simulink model "sym_model copia"  (R2024b)
settings: Solver=FixedStepAuto  StartTime=0  StopTime=24*3600  FixedStep=60  RelTol=1e-3
values from neighbouring files (symbols this model uses):
  FR_consumption = 0*min    [Consumption_profiles.m]
  I_sym = I_feb    [Consumption_profiles.m]
  T_mains = 12    [Consumption_profiles.m]
  Ta_sym = Ta_feb    [Consumption_profiles.m]
  TR_consumption = 0*min    [Consumption_profiles.m]
undefined symbols (not defined in the file or in its folder): A, c, epsilon, eta_zero, m_c, M_s, T_home, tank_LC, Ts_0, U
settings Model: Creator=giacm  LastModifiedBy=edoardomurgia
settings DataIOCC: ReturnWorkspaceOutputs=off
settings DebuggingCC: AlgebraicLoopMsg=none
settings RTWCC: GPUComputeCapability=3.5

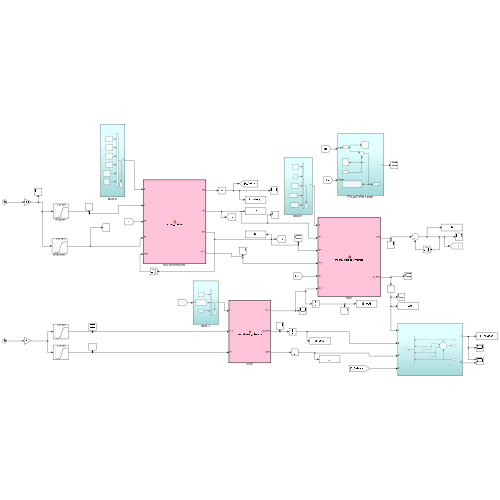
[thumbnail: Simulink's stored preview of the top-level diagram]
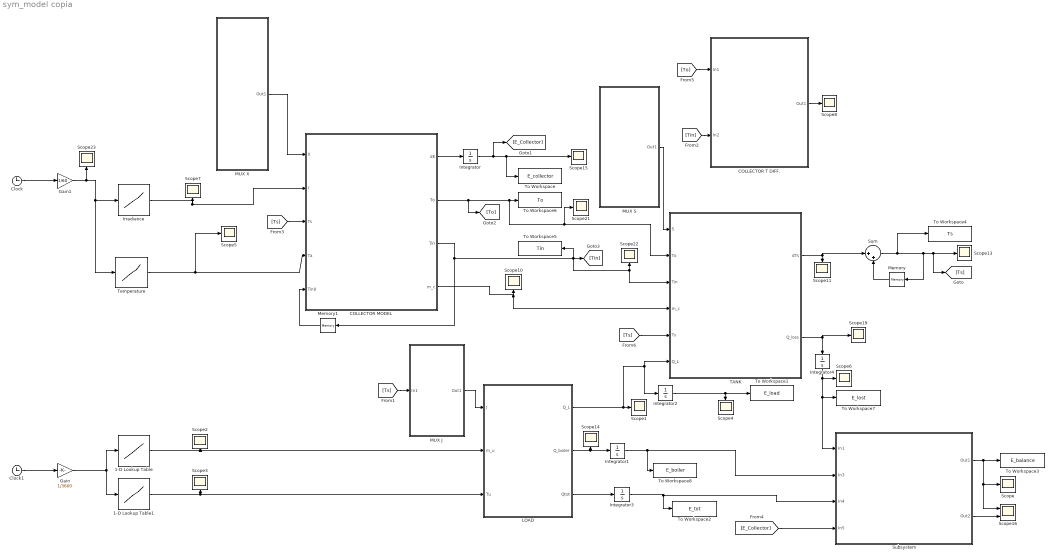
== system sym_model copia ==
  1-D Lookup Table : Lookup_n-D  NumberOfTableDimensions=1  BreakpointsForDimension1=min/60  Table=FR_consumption  InternalRulePriority=Speed  RndMeth=Simplest
  1-D Lookup Table1 : Lookup_n-D  NumberOfTableDimensions=1  BreakpointsForDimension1=min/60  Table=TR_consumption  InternalRulePriority=Speed  RndMeth=Simplest
  COLLECTOR MODEL : MATLAB Function  TreatAsAtomicUnit=on
  COLLECTOR T DIFF. : Subsystem
  Clock : Clock
  Clock1 : Clock
  Gain : Gain  Gain=1/3600
  Gain1 : Gain  Gain=1/60
  Integrator{,1..4} (5 alike) : Integrator
  Irradiance : Lookup_n-D  NumberOfTableDimensions=1  BreakpointsForDimension1=min  Table=I_sym  InternalRulePriority=Speed  RndMeth=Simplest
  LOAD : MATLAB Function  TreatAsAtomicUnit=on
  MUX J : Subsystem
  MUX S : Subsystem
  MUX X : Subsystem
  Memory : Memory  InitialCondition=Ts_0
  Memory1 : Memory  InitialCondition=30
  Scope{,1..8,10..11,13..15,19,21..23} (18 alike) : Scope
  Scope16 : Scope  NumInputPorts=2
  Subsystem : Subsystem
  Sum : Sum  Inputs=|++
  TANK : MATLAB Function  TreatAsAtomicUnit=on
  Temperature : Lookup_n-D  NumberOfTableDimensions=1  BreakpointsForDimension1=min  Table=Ta_sym  InternalRulePriority=Speed  RndMeth=Simplest
  To Workspace : ToWorkspace  VariableName=E_collector  SampleTime=-1
  To Workspace1 : ToWorkspace  VariableName=E_load  SampleTime=-1
  To Workspace2 : ToWorkspace  VariableName=E_tot  SampleTime=-1
  To Workspace3 : ToWorkspace  VariableName=E_balance  SaveFormat=Timeseries  SampleTime=-1
  To Workspace4 : ToWorkspace  VariableName=Ts  SampleTime=-1
  To Workspace5 : ToWorkspace  VariableName=Tin  SampleTime=-1
  To Workspace6 : ToWorkspace  VariableName=To  SampleTime=-1
  To Workspace7 : ToWorkspace  VariableName=E_lost  SampleTime=-1
  To Workspace8 : ToWorkspace  VariableName=E_boiler  SampleTime=-1
  wires:
  1-D Lookup Table/1 -> LOAD/2(m_u), Scope2/1
  1-D Lookup Table1/1 -> LOAD/3(Tu), Scope3/1
  COLLECTOR MODEL/2(To) -> [To], To Workspace6/1, Scope21/1, TANK/2(To)
  Irradiance/1 -> Scope7/1, COLLECTOR MODEL/2(I)
  COLLECTOR MODEL/3(Tin) -> To Workspace5/1, [Tin], TANK/3(Tin), Scope22/1, Memory1/1
  [Ts] -> COLLECTOR MODEL/3(Ts)
  Temperature/1 -> COLLECTOR MODEL/4(Ta), Scope5/1
  Clock1/1 -> Gain/1
  Gain/1 -> 1-D Lookup Table1/1, 1-D Lookup Table/1
  Gain1/1 -> Irradiance/1, Temperature/1, Scope23/1
  Clock/1 -> Gain1/1
  TANK/1(dTs) -> Sum/1, Scope11/1
  Sum/1 -> To Workspace4/1, Scope13/1, [Ts], Memory/1
  COLLECTOR MODEL/4(m_c) -> Scope10/1, TANK/4(m_c)
  COLLECTOR MODEL/1(dE) -> Integrator/1
  Integrator/1 -> Scope15/1, To Workspace/1, [E_Collector]
  LOAD/2(Q_boiler) -> Integrator1/1, Scope14/1
  LOAD/3(Qtot) -> Integrator3/1
  [Ts] -> TANK/5(Ts)
  TANK/2(Q_loss) -> Scope19/1, Integrator4/1
  LOAD/1(Q_L) -> Scope1/1, TANK/6(Q_L), Integrator2/1
  Integrator2/1 -> To Workspace1/1, Scope4/1
  Integrator4/1 -> Scope6/1, Subsystem/1(In1), To Workspace7/1
  Integrator1/1 -> To Workspace8/1, Subsystem/2(In3)
  Integrator3/1 -> Subsystem/3(In4), To Workspace2/1
  [E_Collector] -> Subsystem/4(In5)
  Subsystem/1(Out1) -> Scope/1, Scope16/1, To Workspace3/1
  Subsystem/2(Out2) -> Scope16/2
  Memory/1 -> Sum/2
  Memory1/1 -> COLLECTOR MODEL/5(Tin0)
  [To] -> COLLECTOR T DIFF./1(In1)
  [Tin] -> COLLECTOR T DIFF./2(In2)
  COLLECTOR T DIFF./1(Out1) -> Scope8/1
  MUX S/1(Out1) -> TANK/1(S)
  [Ts] -> MUX J/1(In1)
  MUX J/1(Out1) -> LOAD/1(J)
  MUX X/1(Out1) -> COLLECTOR MODEL/1(X)

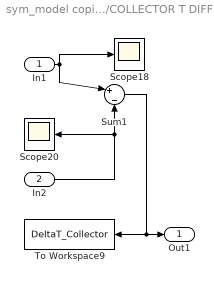
== system sym_model copia/COLLECTOR T DIFF. ==
  In1 : Inport
  In2 : Inport  Port=2
  Scope18 : Scope
  Scope20 : Scope
  Sum1 : Sum  Inputs=|+|-
  To Workspace9 : ToWorkspace  VariableName=DeltaT_Collector  SaveFormat=Timeseries  SampleTime=-1
  Out1 : Outport
  wires:
  In2/1 -> Sum1/2, Scope20/1
  Sum1/1 -> Out1/1, To Workspace9/1
  In1/1 -> Scope18/1, Sum1/1

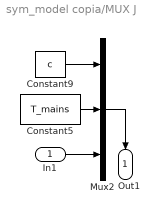
== system sym_model copia/MUX J ==
  In1 : Inport
  Constant5 : Constant  Value=T_mains
  Constant9 : Constant  Value=c
  Mux2 : Mux  Inputs=3
  Out1 : Outport
  wires:
  In1/1 -> Mux2/3
  Mux2/1 -> Out1/1
  Constant9/1 -> Mux2/1
  Constant5/1 -> Mux2/2

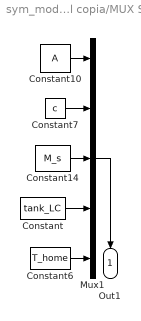
== system sym_model copia/MUX S ==
  Constant : Constant  Value=tank_LC
  Constant10 : Constant  Value=A
  Constant14 : Constant  Value=M_s
  Constant6 : Constant  Value=T_home
  Constant7 : Constant  Value=c
  Mux1 : Mux  Inputs=5
  Out1 : Outport
  wires:
  Mux1/1 -> Out1/1
  Constant/1 -> Mux1/4
  Constant7/1 -> Mux1/2
  Constant10/1 -> Mux1/1
  Constant6/1 -> Mux1/5
  Constant14/1 -> Mux1/3

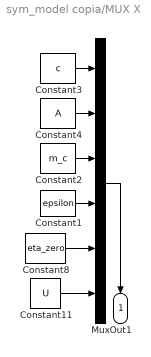
== system sym_model copia/MUX X ==
  Constant1 : Constant  Value=epsilon
  Constant11 : Constant  Value=U
  Constant2 : Constant  Value=m_c
  Constant3 : Constant  Value=c
  Constant4 : Constant  Value=A
  Constant8 : Constant  Value=eta_zero
  Mux : Mux  Inputs=6
  Out1 : Outport
  wires:
  Constant3/1 -> Mux/1
  Constant8/1 -> Mux/5
  Mux/1 -> Out1/1
  Constant4/1 -> Mux/2
  Constant11/1 -> Mux/6
  Constant2/1 -> Mux/3
  Constant1/1 -> Mux/4

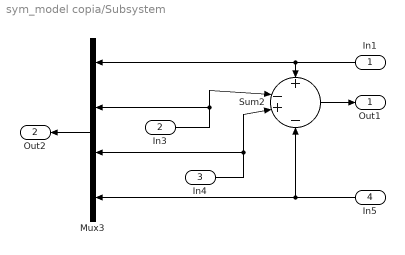
== system sym_model copia/Subsystem ==
  In1 : Inport
  In3 : Inport  Port=2
  In4 : Inport  Port=3
  In5 : Inport  Port=4
  Mux3 : Mux
  Sum2 : Sum  Inputs=+|-+|-
  Out1 : Outport
  Out2 : Outport  Port=2
  wires:
  In5/1 -> Sum2/4, Mux3/4
  Sum2/1 -> Out1/1
  Mux3/1 -> Out2/1
  In4/1 -> Mux3/3, Sum2/3
  In1/1 -> Mux3/1, Sum2/1
  In3/1 -> Mux3/2, Sum2/2

== matlab function sym_model copia/LOAD ==
  data: J input; m_u input; Q_L output; Tu input; Q_boiler output; Qtot output
function [Q_L,Q_boiler,Qtot]  = thermal_energy_balance(J,m_u,Tu)
% MATLAB function to calculate heat losses and boiler contribution
c=J(1);
Tm=J(2);
Ts=J(3);
% Compute Q_L (heat exchange with the storage tank)     4) On the notes
if (Tu <= Ts)
    Q_L = m_u * c * (Tu - Tm);
else
    Q_L = m_u * c * (Ts - Tm);
end

% Compute Q_boiler (boiler activation logic)            5) On the notes
if Tu <= Ts
    Q_boiler = 0;                   % Boiler is not needed
else
    Q_boiler = m_u * c * (Tu - Ts); % Boiler compensates thermal deficit
end
 Qtot= m_u * c * (Tu - Tm);
end

== matlab function sym_model copia/TANK ==
  data: S input; To input; Tin input; m_c input; Ts input; dTs output; Q_L input; Q_loss output
function [dTs,Q_loss] = thermal_storage_dynamics(S,To,Tin,m_c,Ts,Q_L)
A= S(1);
c=S(2);
Ms=S(3);
tank_LC=S(4);
T_home=S(5);
% Compute dTs using the given thermal energy balance equation
Q_loss = tank_LC*A*(Ts-T_home);
% Q_loss=0;
dTs = (m_c * c * (To - Tin) - Q_L -Q_loss ) / (Ms * c);

end

== matlab function sym_model copia/COLLECTOR MODEL ==
  data: X input; I input; Ts input; Ta input; Tin0 input; dE output; To output; Tin output; m_c output
function [dE,To, Tin,m_c] = thermal_collector(X, I, Ts,Ta,Tin0)
% DATA
c= X(1);
A=X(2);
m_c= X(3);
Epsilon= X(4);
eta_zero=X(5);
U=X(6);

if(I<=0)
    eta=0;
else
    eta = eta_zero - (U * ((Tin0 - Ta) / (I)));
end

% From thermal energy balance find To and Tin
To=(A*I*eta + (Ts+273.15)*c*Epsilon*m_c)/(c*Epsilon*m_c)-273.15;
Tin=(A*I*eta - A*I*Epsilon*eta + (Ts+273.15)*c*Epsilon*m_c)/(c*Epsilon*m_c)-273.15;

if( eta < 0 ||I<=0)
   m_c = 0;
end
dE = A*eta*I;

end
